simulink model "MatlabUDPSender"  (R2013a)
settings: Solver=ode4  StartTime=0.0  StopTime=inf  FixedStep=0.1  RelTol=1e-3
libraries: instrumentlib x1
settings Model: Creator=Ssubrama  LastModifiedBy=2049632v
settings DataIOCC: SignalLoggingSaveFormat=ModelDataLogs
settings OptimizationCC: ExpressionDepthLimit=2147483647  InitFltsAndDblsToZero=on
settings DebuggingCC: MultiTaskDSMMsg=warning  MultiTaskCondExecSysMsg=none  FcnCallInpInsideContextMsg=UseLocalSettings  StrictBusMsg=None
settings RTWCC: IncludeERTFirstTime=on
settings GRTTargetCC: TargetFcnLib=ansi_tfl_tmw_new.mat  CodeReplacementLibrary=None  CombineOutputUpdateFcns=off  CPPClassGenCompliant=on  GRTInterface=on

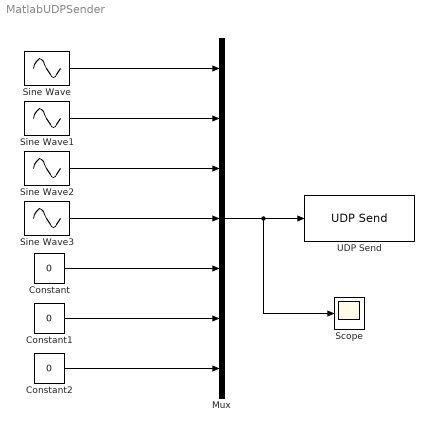
== system MatlabUDPSender ==
  Constant : Constant  Value=0
  Constant1 : Constant  Value=0
  Constant2 : Constant  Value=0
  Mux : Mux  Inputs=7
  Scope : Scope
  Sine Wave : Sin  Priority=1  SampleTime=0.1
  Sine Wave1 : Sin  Priority=1  Bias=4  SampleTime=0.1
  Sine Wave2 : Sin  Priority=1  Bias=-2  SampleTime=0.1
  Sine Wave3 : Sin  Priority=1  Amplitude=2  SampleTime=0.1
  UDP Send : instrumentlib/UDP Send  Priority=2  Host=localhost  Port=51001  LocalPort=51000  EnableBlockingMode=on  ByteOrder=BigEndian
  wires:
  Sine Wave/1 -> Mux/1
  Sine Wave1/1 -> Mux/2
  Sine Wave2/1 -> Mux/3
  Sine Wave3/1 -> Mux/4
  Mux/1 -> Scope/1, UDP Send/1
  Constant/1 -> Mux/5
  Constant1/1 -> Mux/6
  Constant2/1 -> Mux/7
